simulink model "Project5"  (R2014a)
settings: Solver=ode45  StartTime=0.0  StopTime=3600  RelTol=1e-3
values from neighbouring files (symbols this model uses):
  i = 2.3    [Project5_Run.m]
  OCV = Battery_Data(:,2)    [Project5_Run.m]
  Q = 2.3 * 3600    (= 8280)    [Project5_Run.m]
  R_Charging = Battery_Data(:,3)    [Project5_Run.m]
  SOC = Battery_Data(:,1)    [Project5_Run.m]
settings Model: Creator=DZR3QN  LastModifiedBy=DZR3QN

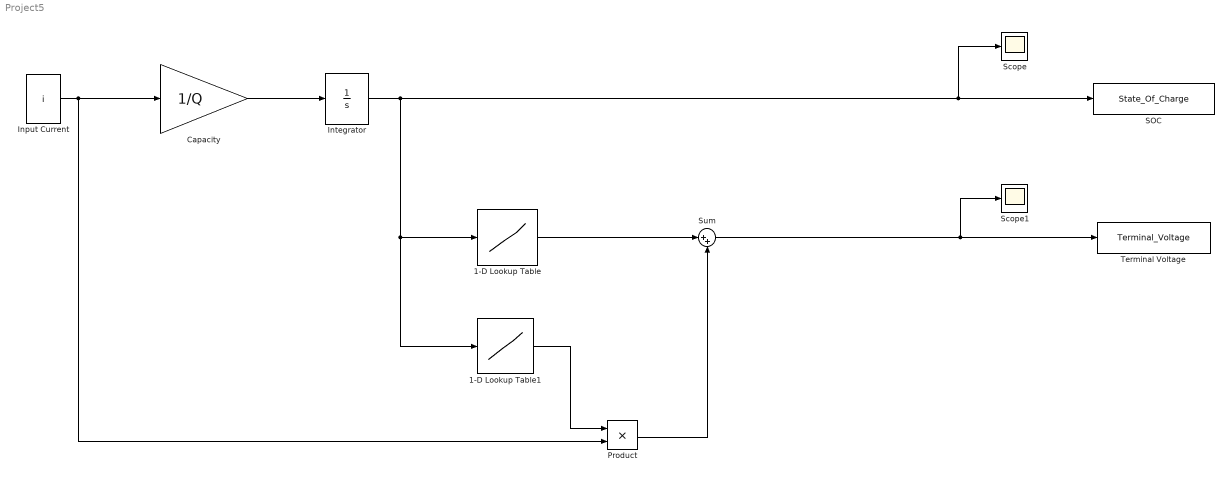
== system Project5 ==
  1-D Lookup Table : Lookup_n-D  NumberOfTableDimensions=1  BreakpointsForDimension1=SOC  Table=OCV  InternalRulePriority=Speed  RndMeth=Simplest  InputSameDT=on
  1-D Lookup Table1 : Lookup_n-D  NumberOfTableDimensions=1  BreakpointsForDimension1=SOC  Table=R_Charging  InternalRulePriority=Speed  RndMeth=Simplest  InputSameDT=on
  Capacity : Gain  Gain=1/Q
  Input Current : Constant  Value=i
  Integrator : Integrator
  Product : Product  RndMeth=Zero
  SOC : ToWorkspace  VariableName=State_Of_Charge  SaveFormat=Structure  SampleTime=-1
  Scope : Scope
  Scope1 : Scope
  Sum : Sum  Inputs=|++
  Terminal Voltage : ToWorkspace  VariableName=Terminal_Voltage  SaveFormat=Structure  SampleTime=-1
  wires:
  Capacity/1 -> Integrator/1
  Input Current/1 -> Product/2, Capacity/1
  Integrator/1 -> 1-D Lookup Table1/1, 1-D Lookup Table/1, Scope/1, SOC/1
  1-D Lookup Table1/1 -> Product/1
  Product/1 -> Sum/2
  1-D Lookup Table/1 -> Sum/1
  Sum/1 -> Scope1/1, Terminal Voltage/1
